simulink model "untitled3"  (R2015a)
settings: Solver=ode45  StartTime=0.0  StopTime=1  RelTol=1e-3
libraries: powerlib x17
settings Model: Creator=MBK  LastModifiedBy=MBK
settings DataIOCC: LimitDataPoints=off

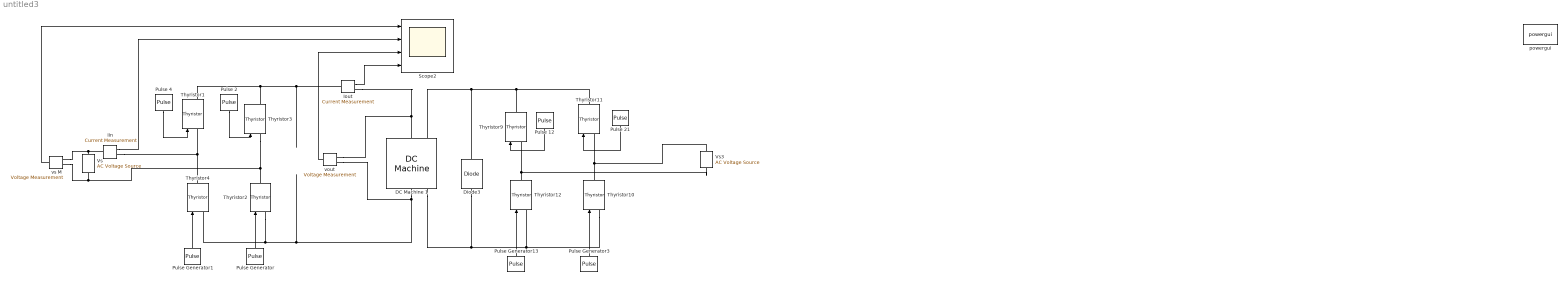
== system untitled3 ==
  DC Machine 1 : powerlib/Machines/DC Machine  PresetModel=No  MechanicalLoad=Speed w  FieldType=Wound  ShowDetailedParameters=on  MeasurementBus=off  RLa="[ 0.6  0.1]"  RLf="[ 240  120]"  Laf=1.8  MachineConstant=Torque constant (N.m/A)  Ke=1.8  Kt=1.8  J=1  Bm=0  Tf=0  w0=1  Ifinit=1  TsPowergui=0  TsBlock=-1
  Diode3 : powerlib/Power Electronics/Diode  Ron=0.001  Lon=0  Vf=0.8  IC=0  UseSnubber=off  Rs=500  Cs=250e-9  Measurements=off
  "Iin " : powerlib/Measurements/Current Measurement  PhasorSimulation=off  OutputType=Complex  PSBequivalent=0
  "Iout " : powerlib/Measurements/Current Measurement  PhasorSimulation=off  OutputType=Complex  PSBequivalent=0
  Pulse 12 : DiscretePulseGenerator  PulseType=Time based  Amplitude=5  Period=0.02  PulseWidth=5  PhaseDelay=60*0.02/360
  Pulse 2 : DiscretePulseGenerator  PulseType=Time based  Amplitude=5  Period=0.02  PulseWidth=5  PhaseDelay=240*0.02/360
  Pulse 21 : DiscretePulseGenerator  PulseType=Time based  Amplitude=5  Period=0.02  PulseWidth=5  PhaseDelay=240*0.02/360
  Pulse 4 : DiscretePulseGenerator  PulseType=Time based  Amplitude=5  Period=0.02  PulseWidth=5  PhaseDelay=60*0.02/360
  Pulse Generator : DiscretePulseGenerator  PulseType=Time based  Amplitude=5  Period=0.02  PulseWidth=5  PhaseDelay=60*0.02/360
  Pulse Generator1 : DiscretePulseGenerator  PulseType=Time based  Amplitude=5  Period=0.02  PulseWidth=5  PhaseDelay=240*0.02/360
  Pulse Generator13 : DiscretePulseGenerator  PulseType=Time based  Amplitude=5  Period=0.02  PulseWidth=5  PhaseDelay=240*0.02/360
  Pulse Generator3 : DiscretePulseGenerator  PulseType=Time based  Amplitude=5  Period=0.02  PulseWidth=5  PhaseDelay=60*0.02/360
  Scope2 : Scope  NumInputPorts=4
      settings: YMin=-5~-5~-5~-5  YMax=5~5~5~5
  Thyristor1 : powerlib/Power Electronics/Thyristor  Ron=0.001  Lon=0  Vf=0.8  IC=0  Rs=500  Cs=250e-9  Measurements=on
  Thyristor{2,4,9..12} (6 alike) : powerlib/Power Electronics/Thyristor  Ron=0.001  Lon=0  Vf=0.8  IC=0  Rs=500  Cs=250e-9  Measurements=off
  Thyristor3 : powerlib/Power Electronics/Thyristor  Ron=0.001  Lon=0  Vf=0.8  IC=0  Rs=500  Cs=250e-9  Measurements=on
  "Vs " : powerlib/Electrical Sources/AC Voltage Source  Amplitude=220*sqrt(2)  Phase=0  Frequency=50  SampleTime=0  Measurements=None
  Vs3 : powerlib/Electrical Sources/AC Voltage Source  Amplitude=220*sqrt(2)  Phase=0  Frequency=50  SampleTime=0  Measurements=None
  powergui : powerlib/powergui  Priority=1  SimulationMode=Continuous  SolverType=Tustin/Backward Euler (TBE)  SampleTime=50e-6  frequency=60  SPID=off  DisableSnubberDevices=off  DisableRonSwitches=off  DisableVfSwitches=off  SwTol=0  DisplayEquations=off  Interpol=off  methode=off  Ts=100  FunctionMessages=off  echomessages=off  HookPort=off  EnableUseOfTLC=off  x0status=blocks  frequencyindice=0  Pbase=100e6  ErrMax=1e-4  Iterations=50  UnitsV=kV  UnitsW=MW  buscounter=0  RestoreLinks=warning  ResistiveCurrentMeasurement=off  Frange=[0:2:500]  Ylog=off  Xlog=on  ShowGrid=off  save=off  variable=ZData  structure=0  ZoomFFT=off  StartTime=0.0  cycles=1  DisplayStyle=1  fundamental=60  FreqAxis=off  MaxFrequency=1000  frequencyindicesteady=1  RmsSteady=1  display=off
  "vout " : powerlib/Measurements/Voltage Measurement  PhasorSimulation=off  OutputType=Complex  PSBequivalent=0
  "vs M " : powerlib/Measurements/Voltage Measurement  PhasorSimulation=off  OutputType=Complex  PSBequivalent=0
  wires:
  Pulse Generator/1 -> Thyristor2/1
  "vs M "/1 -> Scope2/1
  "Iin "/1 -> Scope2/2
  "Iout "/1 -> Scope2/4
  Pulse Generator1/1 -> Thyristor4/1
  Pulse Generator13/1 -> Thyristor12/1
  "vout "/1 -> Scope2/3
  Pulse 4/1 -> Thyristor1/1
  Pulse 2/1 -> Thyristor3/1
  Pulse Generator3/1 -> Thyristor10/1
  Pulse 12/1 -> Thyristor9/1
  Pulse 21/1 -> Thyristor11/1
  connections:
  Thyristor4/RConn1 -- "Iin "/RConn1 -- Thyristor1/LConn1
  Thyristor3/LConn1 -- "vs M "/LConn2 -- "Vs "/LConn1 -- Thyristor2/RConn1
  Thyristor1/RConn1 -- "Iout "/LConn1 -- Thyristor3/RConn1
  Thyristor2/LConn1 -- Thyristor4/LConn1 -- DC Machine 1/RConn1 -- "vout "/LConn2
  Thyristor11/LConn1 -- Vs3/RConn1 -- Thyristor10/RConn1
  Vs3/LConn1 -- Thyristor12/RConn1 -- Thyristor9/LConn1
  Thyristor11/RConn1 -- DC Machine 1/LConn2 -- Diode3/RConn1 -- Thyristor9/RConn1
  Thyristor10/LConn1 -- DC Machine 1/RConn2 -- Diode3/LConn1 -- Thyristor12/LConn1
  "Iin "/LConn1 -- "Vs "/RConn1 -- "vs M "/LConn1
  "Iout "/RConn1 -- "vout "/LConn1 -- DC Machine 1/LConn1
